simulink model "lab4"  (R2018b)
settings: Solver=ode45  StartTime=0.0  StopTime=10.0  MaxStep=2^-5  RelTol=1e-3
libraries: simulink x1
settings Model: Creator=vandavv  LastModifiedBy=vandavv

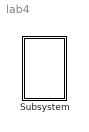
== system lab4 ==
  Subsystem : Subsystem  mask{g=9.81, m1=1, m2=3, M=1, R=0.001, r0=1, f0=90}

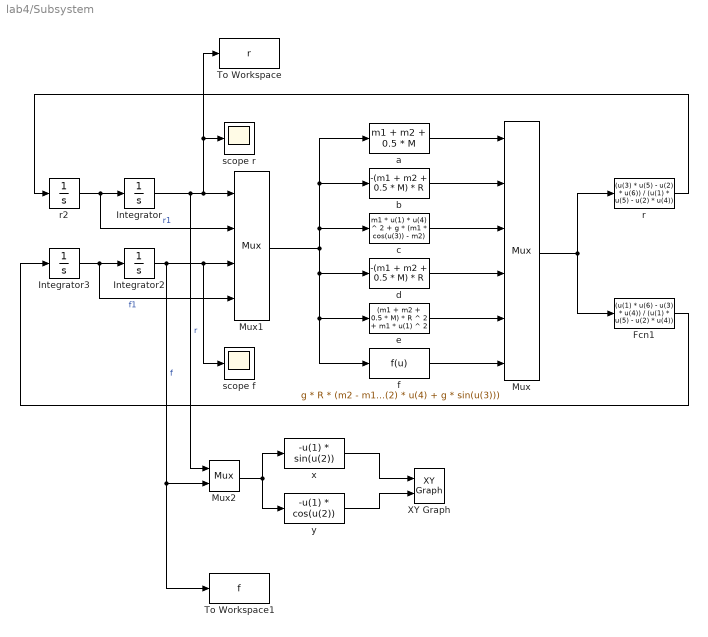
== system lab4/Subsystem ==
  Fcn1 : Fcn  Expr=(u(1) * u(6) - u(3) * u(4)) / (u(1) * u(5) - u(2) * u(4))
  Integrator : Integrator  InitialCondition=r0
  Integrator2 : Integrator  InitialCondition=f0 * pi / 180
  Integrator3 : Integrator
  Mux : Mux  Inputs=6
  Mux1 : Mux
  Mux2 : Mux  Inputs=2
  To Workspace : ToWorkspace  VariableName=r  SampleTime=-1
  To Workspace1 : ToWorkspace  VariableName=f  SampleTime=-1
  XY Graph : simulink/Sinks/XY Graph  xmin=-2  xmax=2  ymin=-2  ymax=2  st=-1
  a : Fcn  Expr=m1 + m2 + 0.5 * M
  b : Fcn  Expr=-(m1 + m2 + 0.5 * M) * R
  c : Fcn  Expr="m1  * u(1) * u(4) ^ 2 + g * (m1 * cos(u(3)) - m2)"
  d : Fcn  Expr=-(m1 + m2 + 0.5 * M) * R
  e : Fcn  Expr=(m1 + m2 + 0.5 * M) * R ^ 2 + m1 * u(1) ^ 2
  f : Fcn  Expr=g * R * (m2 - m1 * cos(u(3))) - m1 * u(1) * (2 * u(2) * u(4) + g * sin(u(3)))
  r : Fcn  Expr=(u(3) * u(5) - u(2) * u(6)) / (u(1) * u(5) - u(2) * u(4))
  r2 : Integrator
  scope f : Scope
  scope r : Scope
  x : Fcn  Expr=-u(1) * sin(u(2))
  y : Fcn  Expr=-u(1) * cos(u(2))
  wires:
  a/1 -> Mux/1
  b/1 -> Mux/2
  r/1 -> r2/1
  Fcn1/1 -> Integrator3/1
  Mux/1 -> Fcn1/1, r/1
  e/1 -> Mux/5
  d/1 -> Mux/4
  Integrator3/1 -> Mux1/4, Integrator2/1  "f1"
  f/1 -> Mux/6
  Mux1/1 -> d/1, e/1, f/1, a/1, b/1, c/1
  r2/1 -> Mux1/2, Integrator/1  "r1"
  c/1 -> Mux/3
  Integrator/1 -> Mux2/1, To Workspace/1, scope r/1, Mux1/1  "r"
  Integrator2/1 -> To Workspace1/1, Mux2/2, scope f/1, Mux1/3  "f"
  Mux2/1 -> y/1, x/1
  x/1 -> XY Graph/1
  y/1 -> XY Graph/2
